simulink model "lab_6"  (Simulink 7.3)
settings: Solver=ode3  StartTime=0.0  StopTime=100  FixedStep=0.001  RelTol=1e-3
libraries: simulink x3
settings Model: Creator=torres.g  LastModifiedBy=torres.g

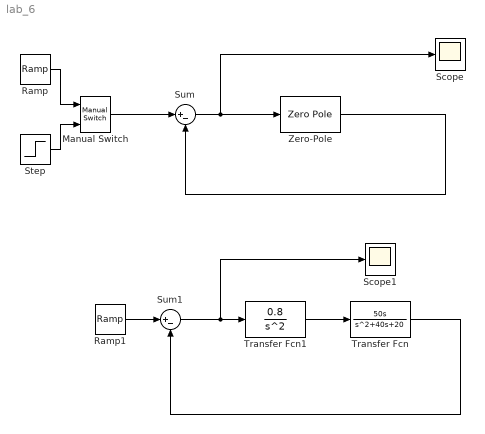
== system lab_6 ==
  Manual Switch : simulink/Signal Routing/Manual Switch  SystemSampleTime=-1  sw=1  action=0  varsize=off
  Ramp : simulink/Sources/Ramp  SystemSampleTime=-1  slope=5  start=0  X0=0
  Ramp1 : simulink/Sources/Ramp  SystemSampleTime=-1  slope=1  start=0  X0=0
  Scope : Scope
      settings: YMin=1.6  YMax=1.6
  Scope1 : Scope
      settings: YMin=1.52  YMax=1.68
  Step : Step  Time=0  After=5  SampleTime=0
  Sum : Sum  Inputs=|+-  OutDataType=fixdt(1, 16)  OutScaling=2^0
  Sum1 : Sum  Inputs=|+-  OutDataType=fixdt(1, 16)  OutScaling=2^0
  Transfer Fcn : TransferFcn  Numerator=[50 0]  Denominator=[1 40 20]
  Transfer Fcn1 : TransferFcn  Numerator=[0.8]  Denominator=[1 0 0]
  Zero-Pole : ZeroPole  Zeros=[-1 -5]  Poles=[0 -2 -8]  Gain=[10]
  wires:
  Sum/1 -> Zero-Pole/1, Scope/1
  Zero-Pole/1 -> Sum/2
  Ramp1/1 -> Sum1/1
  Transfer Fcn/1 -> Sum1/2
  Sum1/1 -> Transfer Fcn1/1, Scope1/1
  Transfer Fcn1/1 -> Transfer Fcn/1
  Ramp/1 -> Manual Switch/1
  Step/1 -> Manual Switch/2
  Manual Switch/1 -> Sum/1
